simulink model "OFDM_Rx_HW"  (R2020a)
settings: Solver=FixedStepDiscrete  StartTime=0.0  StopTime=inf  RelTol=1e-3
InitFcn:
  | % Set parameters
  | fs = 1e6;
  | 
  | % Load all required variables
  | load('variables/read_addr_data');
  | load('variables/read_addr_cp');
  | load('variables/read_addr_pream');
  | load('variables/read_addr_rx');
  | load('variables/pilot');
  | load('variables/sc_index');
  | load('variables/LTSfreq');
  | load('variables/STSfreq');
  | load('variables/LTSread');
  | load('variables/STSread');
  | 
  | run ./scripts/rfgen;
undefined symbols (not defined in the file or in its folder): LTSfreq, LTSread, pilot, read_addr_cp, read_addr_data, read_addr_pream, read_addr_rx, sc_index, STSfreq, STSread
libraries: hdlsllib x78, simulink x55, xbsIndex_r4 x22, dspmlti4 x19, dspsigops x6, dsphdlmathfun x3, dsphdlxfrm x2, dsphdlsigops x1, lib_rfsignalgenerator x1
(part 1 of 4)
settings Model: SimulationMode=accelerator  Creator=njb13206  LastModifiedBy=david
settings OptimizationCC: BlockReduction=off  ConditionallyExecuteInputs=off  DefaultParameterBehavior=Inlined
settings DebuggingCC: AlgebraicLoopMsg=error  SingleTaskRateTransMsg=error  IntegerOverflowMsg=none  ParameterPrecisionLossMsg=none  IntegerSaturationMsg=none
settings HardwareCC: ProdBitPerPointer=32  ProdBitPerSizeT=32  ProdBitPerPtrDiffT=32  ProdLargestAtomicFloat=None  ProdIntDivRoundTo=Undefined  ProdEndianess=Unspecified  ProdWordSize=32  ProdHWDeviceType=ASIC/FPGA->ASIC/FPGA  TargetBitPerPointer=64  TargetBitPerSizeT=64  TargetBitPerPtrDiffT=64  TargetLongLongMode=on  TargetIntDivRoundTo=Zero  TargetEndianess=LittleEndian  TargetWordSize=64  TargetHWDeviceType=Custom Processor->MATLAB Host Computer  ProdEqTarget=off

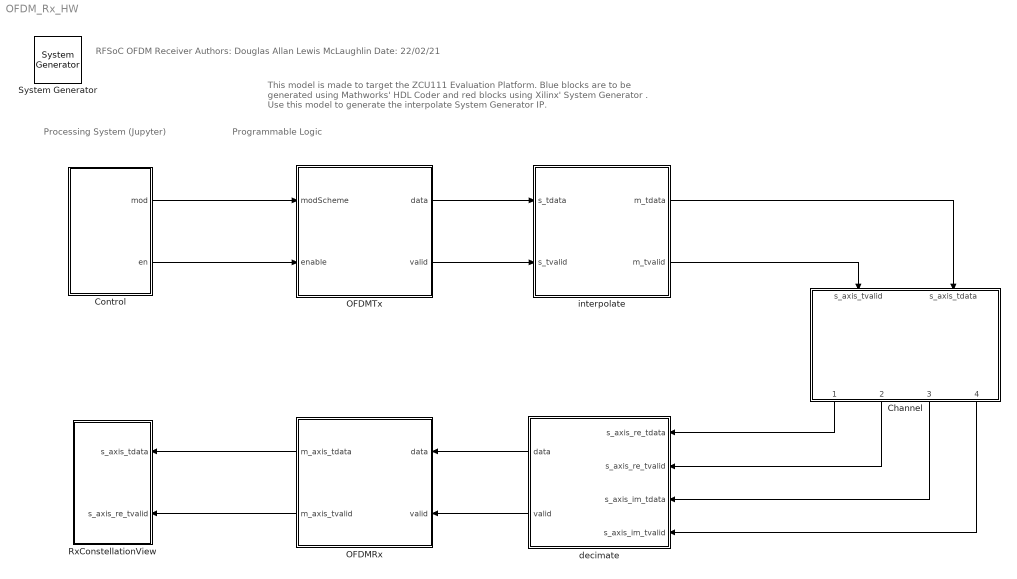
== system OFDM_Rx_HW ==
  note: This model is made to target the ZCU111 Evaluation Platform. Blue blocks are to be generated using Mathworks' HDL Coder and red blocks using Xilinx' System Generator .
      |
      | Use this model to generate the interpolate System Generator IP.
  note: Programmable Logic
  note: Processing System (Jupyter)
  note: RFSoC OFDM Receiver
      | Authors: Douglas Allan
      | Lewis McLaughlin
      | Date: 22/02/21
  " System Generator" : xbsIndex_r4/ System Generator  Tag=genX  xilinxfamily=zynquplusRFSOC  part=xczu28dr  speed=-2-e  package=ffvg1517  synthesis_tool=Vivado  clock_wrapper=Clock Enables  directory=./netlist  proj_type=Vivado  Synth_file=Vivado Synthesis Defaults  Impl_file=Vivado Implementation Defaults  testbench=off  simulink_period=1/256e6  sysclk_period=(1/256e6)*1e9  dcm_input_clock_period=10  incr_netlist=off  trim_vbits=Everywhere in SubSystem  dbl_ovrd=According to Block Masks  core_generation=According to Block Masks  run_coregen=off  deprecated_control=off  eval_field=0  block_type=sysgen
  Channel : Subsystem
  Control : Subsystem  mask{mod_mask=64QAM, en=on}
      mask prompts: mod_mask "Modulation"; en "Enable"
      mask init:
      | % RF Signal Generator
      | if strcmpi(get_param(gcb, 'mod_mask'), 'BPSK')
      |     mod = 0;
      | elseif strcmpi(get_param(gcb, 'mod_mask'), 'QPSK')
      |     mod = 1;
      | elseif strcmpi(get_param(gcb, 'mod_mask'), '8PSK')
      |     mod = 2;
      | elseif strcmpi(get_param(gcb, 'mod_mask'), '16QAM')
      |     mod = 3;
      | elseif strcmpi(get_param(gcb, 'mod_mask'), '32QAM')
      |     mod = 4;
      | elseif strcmpi(get_param(gcb, 'mod_mask'), '64QAM')
      |     mod = 5;
      | elseif strcmpi(get_param(gcb, 'mod_mask'), '128QAM')
      |     mod = 6;
      | elseif strcmpi(get_param(gcb, 'mod_mask'), '256QAM')
      |     mod = 7;
      | elseif strcmpi(get_param(gcb, 'mod_mask'), '512QAM')
      |     mod = 8;
      | elseif strcmpi(get_param(gcb, 'mod_mask'), '1024QAM')
      |     mod = 9;
      | end
      mask TypeOptions mod_mask: BPSK | QPSK | 8PSK | 16QAM | 32QAM | 64QAM | 128QAM | 256QAM | 512QAM | 1024QAM
      mask DialogControl DescGroupVar Prompt: RF Signal Generator
      mask DialogControl DescTextVar Prompt: Exposes parameters the user can control from Jupyter when running on the target.
      mask DialogControl Container3 Prompt: Control
  OFDMRx : Subsystem  TreatAsAtomicUnit=on
  OFDMTx : Subsystem  TreatAsAtomicUnit=on
  RxConstellationView : Subsystem
  decimate : Subsystem
  interpolate : Subsystem
  wires:
  interpolate/1(m_tdata) -> Channel/2(s_axis_tdata)
  OFDMTx/1(data) -> interpolate/1(s_tdata)
  OFDMTx/2(valid) -> interpolate/2(s_tvalid)
  interpolate/2(m_tvalid) -> Channel/1(s_axis_tvalid)
  Channel/4(m_axis_im_tvalid) -> decimate/4(s_axis_im_tvalid)
  OFDMRx/1(m_axis_tdata) -> RxConstellationView/1(s_axis_tdata)
  OFDMRx/2(m_axis_tvalid) -> RxConstellationView/2(s_axis_re_tvalid)
  Channel/1(m00_axis_re_tdata) -> decimate/1(s_axis_re_tdata)
  Channel/2(m_axis_re_tvalid) -> decimate/2(s_axis_re_tvalid)
  Channel/3(m01_axis_im_tdata) -> decimate/3(s_axis_im_tdata)
  decimate/2(valid) -> OFDMRx/2(valid)
  decimate/1(data) -> OFDMRx/1(data)
  Control/1(mod) -> OFDMTx/1(modScheme)
  Control/2(en) -> OFDMTx/2(enable)

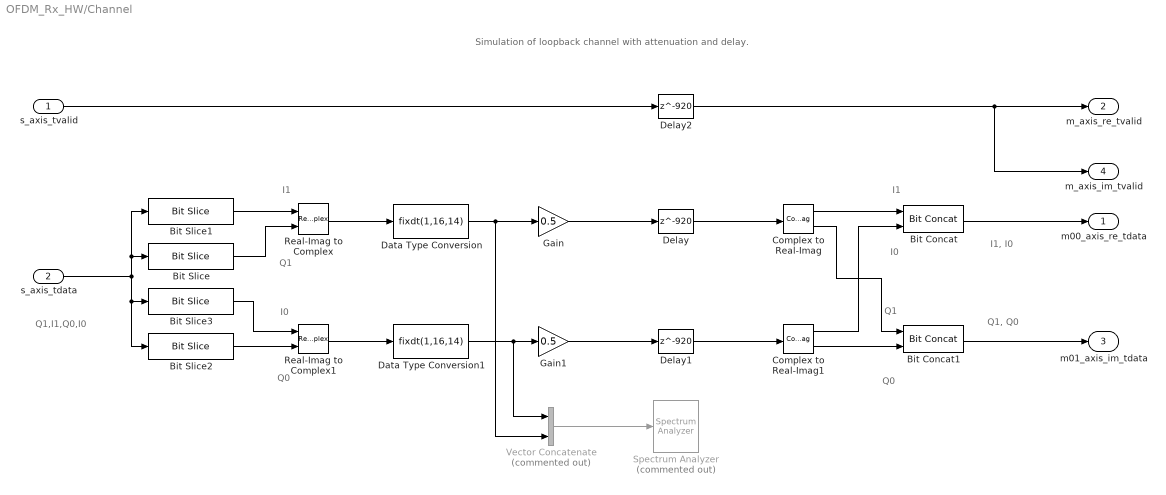
== system OFDM_Rx_HW/Channel ==
  note: Q1, Q0
  note: I1, I0
  note: Q0
  note: I0
  note: Q1
  note: I1
  note: Q1,I1,Q0,I0
  note: Simulation of loopback channel with attenuation and delay.
  note: I1
  note: I0
  note: Q1
  note: Q0
  s_axis_tvalid : Inport
  s_axis_tdata : Inport  Port=2
  Bit Concat : hdlsllib/Logic and Bit Operations/Bit Concat  numInputs=2
  Bit Concat1 : hdlsllib/Logic and Bit Operations/Bit Concat  numInputs=2
  Bit Slice : hdlsllib/Logic and Bit Operations/Bit Slice  lidx=63  ridx=48
      settings: SourceProductBaseCode=SL
  Bit Slice1 : hdlsllib/Logic and Bit Operations/Bit Slice  lidx=47  ridx=32
      settings: SourceProductBaseCode=SL
  Bit Slice2 : hdlsllib/Logic and Bit Operations/Bit Slice  lidx=31  ridx=16
      settings: SourceProductBaseCode=SL
  Bit Slice3 : hdlsllib/Logic and Bit Operations/Bit Slice  lidx=15  ridx=0
      settings: SourceProductBaseCode=SL
  Complex to Real-Imag : ComplexToRealImag
  Complex to Real-Imag1 : ComplexToRealImag
  Data Type Conversion : DataTypeConversion  OutDataTypeStr=fixdt(1,16,14)  ConvertRealWorld=Stored Integer (SI)
  Data Type Conversion1 : DataTypeConversion  OutDataTypeStr=fixdt(1,16,14)  ConvertRealWorld=Stored Integer (SI)
  Delay : Delay  DelayLength=920
  Delay1 : Delay  DelayLength=920
  Delay2 : Delay  DelayLength=920
  Gain : Gain  Gain=0.5  ParamDataTypeStr=double  OutDataTypeStr=fixdt(1,16,14)
  Gain1 : Gain  Gain=0.5  ParamDataTypeStr=double  OutDataTypeStr=fixdt(1,16,14)
  Real-Imag to Complex : RealImagToComplex
  Real-Imag to Complex1 : RealImagToComplex
  Spectrum Analyzer : SpectrumAnalyzer  Commented=on
  Vector Concatenate : Concatenate  Commented=on
  m00_axis_re_tdata : Outport  VectorParamsAs1DForOutWhenUnconnected=off
  m_axis_re_tvalid : Outport  Port=2  VectorParamsAs1DForOutWhenUnconnected=off
  m01_axis_im_tdata : Outport  Port=3  VectorParamsAs1DForOutWhenUnconnected=off
  m_axis_im_tvalid : Outport  Port=4  VectorParamsAs1DForOutWhenUnconnected=off
  wires:
  Gain/1 -> Delay/1
  s_axis_tvalid/1 -> Delay2/1
  Delay/1 -> Complex to Real-Imag/1
  s_axis_tdata/1 -> Bit Slice1/1, Bit Slice/1, Bit Slice2/1, Bit Slice3/1
  Delay1/1 -> Complex to Real-Imag1/1
  Gain1/1 -> Delay1/1
  Bit Concat/1 -> m00_axis_re_tdata/1
  Bit Concat1/1 -> m01_axis_im_tdata/1
  Bit Slice/1 -> Real-Imag to Complex/2
  Bit Slice1/1 -> Real-Imag to Complex/1
  Bit Slice2/1 -> Real-Imag to Complex1/2
  Bit Slice3/1 -> Real-Imag to Complex1/1
  Real-Imag to Complex/1 -> Data Type Conversion/1
  Real-Imag to Complex1/1 -> Data Type Conversion1/1
  Complex to Real-Imag1/1 -> Bit Concat/2
  Complex to Real-Imag/1 -> Bit Concat/1
  Complex to Real-Imag1/2 -> Bit Concat1/2
  Complex to Real-Imag/2 -> Bit Concat1/1
  Data Type Conversion/1 -> Vector Concatenate/2, Gain/1
  Data Type Conversion1/1 -> Vector Concatenate/1, Gain1/1
  Delay2/1 -> m_axis_re_tvalid/1, m_axis_im_tvalid/1
  Vector Concatenate/1 -> Spectrum Analyzer/1

== system OFDM_Rx_HW/Control ==
  Constant2 : Constant  Value=en  OutDataTypeStr=boolean  SampleTime=1/(fs)
  Constant7 : Constant  Value=mod  VectorParams1D=off  OutDataTypeStr=uint32  SampleTime=1/(fs)
  Delay : Delay  DelayLength=randi(10)
  Delay3 : Delay  DelayLength=randi(10)
  mod : Outport  VectorParamsAs1DForOutWhenUnconnected=off
  en : Outport  Port=2  VectorParamsAs1DForOutWhenUnconnected=off
  wires:
  Constant2/1 -> Delay3/1
  Constant7/1 -> Delay/1
  Delay/1 -> mod/1
  Delay3/1 -> en/1

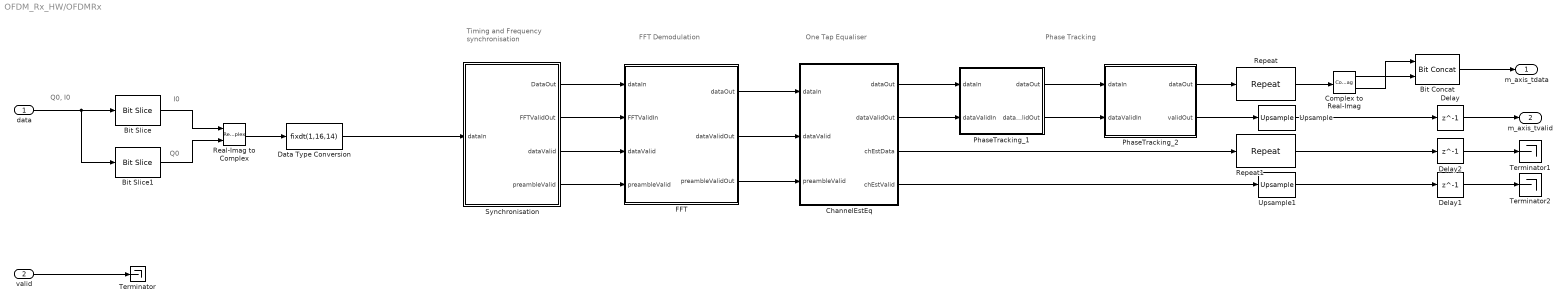
== system OFDM_Rx_HW/OFDMRx ==
  note: Phase Tracking
  note: One Tap Equaliser
  note: FFT Demodulation
  note: Timing and Frequency
      | synchronisation
  note: Q0, I0
  note: I0
  note: Q0
  data : Inport
  valid : Inport  Port=2
  Bit Concat : hdlsllib/Logic and Bit Operations/Bit Concat  numInputs=2
  Bit Slice : hdlsllib/Logic and Bit Operations/Bit Slice  lidx=15  ridx=0
      settings: SourceProductBaseCode=SL
  Bit Slice1 : hdlsllib/Logic and Bit Operations/Bit Slice  lidx=31  ridx=16
      settings: SourceProductBaseCode=SL
  ChannelEstEq : Subsystem
  Complex to Real-Imag : ComplexToRealImag
  Data Type Conversion : DataTypeConversion  OutDataTypeStr=fixdt(1,16,14)  ConvertRealWorld=Stored Integer (SI)
  Delay : Delay  DelayLength=1
  Delay1 : Delay  DelayLength=1
  Delay2 : Delay  DelayLength=1
  FFT : Subsystem
  PhaseTracking_1 : Subsystem
  PhaseTracking_2 : Subsystem
  Real-Imag to Complex : RealImagToComplex
  Repeat : dspsigops/Repeat  N=256  InputProcessing=Columns as channels (frame based)  RateOptions=Allow multirate processing  ic=0  mode=Unused parameter value
  Repeat1 : dspsigops/Repeat  N=256  InputProcessing=Columns as channels (frame based)  RateOptions=Allow multirate processing  ic=0  mode=Unused parameter value
  Synchronisation : Subsystem
  Terminator : Terminator
  Terminator1 : Terminator
  Terminator2 : Terminator
  Upsample : dspsigops/Upsample  N=256  phase=5  RateOptions=Allow multirate processing  ic=0  mode=Unused parameter value
  Upsample1 : dspsigops/Upsample  N=256  phase=5  RateOptions=Allow multirate processing  ic=0  mode=Unused parameter value
  m_axis_tdata : Outport  VectorParamsAs1DForOutWhenUnconnected=off
  m_axis_tvalid : Outport  Port=2  VectorParamsAs1DForOutWhenUnconnected=off
  wires:
  Delay/1 -> m_axis_tvalid/1
  Upsample/1 -> Delay/1
  valid/1 -> Terminator/1
  data/1 -> Bit Slice/1, Bit Slice1/1
  Bit Slice1/1 -> Real-Imag to Complex/2
  Bit Slice/1 -> Real-Imag to Complex/1
  Bit Concat/1 -> m_axis_tdata/1
  Complex to Real-Imag/1 -> Bit Concat/2
  Complex to Real-Imag/2 -> Bit Concat/1
  Repeat/1 -> Complex to Real-Imag/1
  PhaseTracking_2/2(validOut) -> Upsample/1
  PhaseTracking_2/1(dataOut) -> Repeat/1
  Data Type Conversion/1 -> Synchronisation/1(dataIn)
  Real-Imag to Complex/1 -> Data Type Conversion/1
  FFT/1(dataOut) -> ChannelEstEq/1(dataIn)
  FFT/3(preambleValidOut) -> ChannelEstEq/3(preambleValid)
  FFT/2(dataValidOut) -> ChannelEstEq/2(dataValid)
  Synchronisation/1(DataOut) -> FFT/1(dataIn)
  Synchronisation/2(FFTValidOut) -> FFT/2(FFTValidIn)
  Synchronisation/3(dataValid) -> FFT/3(dataValid)
  Synchronisation/4(preambleValid) -> FFT/4(preambleValid)
  ChannelEstEq/1(dataOut) -> PhaseTracking_1/1(dataIn)
  ChannelEstEq/2(dataValidOut) -> PhaseTracking_1/2(dataValidIn)
  PhaseTracking_1/1(dataOut) -> PhaseTracking_2/1(dataIn)
  PhaseTracking_1/2(dataValidOut) -> PhaseTracking_2/2(dataValidIn)
  Upsample1/1 -> Delay1/1
  ChannelEstEq/4(chEstValid) -> Upsample1/1
  ChannelEstEq/3(chEstData) -> Repeat1/1
  Repeat1/1 -> Delay2/1
  Delay2/1 -> Terminator1/1
  Delay1/1 -> Terminator2/1

== system OFDM_Rx_HW/OFDMTx ==
  note: Generate random integers, M-QAM symbol mapping and sub-carrier
      | mapping.
  note: Add Cyclic Prefix
  note: Create OFDM symbols using
      | IFFT
  modScheme : Inport
  enable : Inport  Port=2
  Bit Concat : hdlsllib/Logic and Bit Operations/Bit Concat  numInputs=2
  Bit Slice : hdlsllib/Logic and Bit Operations/Bit Slice  lidx=0  ridx=0
      settings: SourceProductBaseCode=SL
  CPAdd : Subsystem
  Complex to Real-Imag : ComplexToRealImag
  Constant : Constant  OutDataTypeStr=boolean  SampleTime=1/fs
  ControlSignalGenerator : Subsystem
  Data Type Conversion : DataTypeConversion  OutDataTypeStr=uint16  ConvertRealWorld=Stored Integer (SI)
  Data Type Conversion1 : DataTypeConversion  OutDataTypeStr=uint16  ConvertRealWorld=Stored Integer (SI)
  Data Type Conversion2 : DataTypeConversion  OutDataTypeStr=boolean  ConvertRealWorld=Stored Integer (SI)
  DataGenerator : Subsystem
  IFFT : Subsystem
  SCMapper : Subsystem
  Terminator : Terminator
  data : Outport  VectorParamsAs1DForOutWhenUnconnected=off
  valid : Outport  Port=2  VectorParamsAs1DForOutWhenUnconnected=off
  wires:
  Bit Slice/1 -> Data Type Conversion2/1
  enable/1 -> Bit Slice/1
  Data Type Conversion/1 -> Bit Concat/2
  Data Type Conversion1/1 -> Bit Concat/1
  Complex to Real-Imag/2 -> Data Type Conversion1/1
  Complex to Real-Imag/1 -> Data Type Conversion/1
  Bit Concat/1 -> data/1
  modScheme/1 -> DataGenerator/1(modScheme)
  DataGenerator/1(dataOut) -> SCMapper/1(dataIn)
  DataGenerator/2(preambValOut) -> SCMapper/2(preambValid)
  DataGenerator/3(dataValidOut) -> SCMapper/3(dataValid)
  SCMapper/1(dataOut) -> IFFT/1(dataIn)
  SCMapper/2(preambValidOut) -> IFFT/2(preambleValidIn)
  SCMapper/3(dataValidOut) -> IFFT/3("dataValidIn ")
  IFFT/1(dataOut) -> CPAdd/1(dataIn)
  IFFT/2(preambValidOut) -> CPAdd/2(preambValid)
  IFFT/3(dataValidOut) -> CPAdd/3(dataValid)
  CPAdd/1(dataOut) -> Complex to Real-Imag/1
  ControlSignalGenerator/1(dataValid) -> DataGenerator/2(dataValid)
  ControlSignalGenerator/2(preambleValid) -> DataGenerator/3(preambleValid)
  ControlSignalGenerator/3(dataReady) -> DataGenerator/4(dataReady)
  ControlSignalGenerator/4(PilotValid) -> DataGenerator/5(pilotValid)
  Data Type Conversion2/1 -> ControlSignalGenerator/1(enable)
  Constant/1 -> valid/1
  DataGenerator/4(symValidOut) -> Terminator/1

== system OFDM_Rx_HW/RxConstellationView ==
  s_axis_tdata : Inport
  s_axis_re_tvalid : Inport  Port=2
  Bit Slice : hdlsllib/Logic and Bit Operations/Bit Slice  lidx=15  ridx=0
      settings: SourceProductBaseCode=SL
  Bit Slice1 : hdlsllib/Logic and Bit Operations/Bit Slice  lidx=31  ridx=16
      settings: SourceProductBaseCode=SL
  Constant : Constant  Value=NaN + 1i*NaN  OutDataTypeStr=double  SampleTime=-1
  Constellation Diagram : ConstellationDiagram
  Data Type Conversion : DataTypeConversion  OutDataTypeStr=fixdt(1,16,14)  ConvertRealWorld=Stored Integer (SI)
  Real-Imag to Complex : RealImagToComplex
  Switch : Switch  Criteria=u2 ~= 0
  wires:
  Switch/1 -> Constellation Diagram/1
  Constant/1 -> Switch/3
  s_axis_re_tvalid/1 -> Switch/2
  Real-Imag to Complex/1 -> Data Type Conversion/1
  Bit Slice/1 -> Real-Imag to Complex/1
  s_axis_tdata/1 -> Bit Slice1/1, Bit Slice/1
  Bit Slice1/1 -> Real-Imag to Complex/2
  Data Type Conversion/1 -> Switch/1

== system OFDM_Rx_HW/decimate ==
  s_axis_re_tdata : Inport
  s_axis_re_tvalid : Inport  Port=2
  s_axis_im_tdata : Inport  Port=3
  s_axis_im_tvalid : Inport  Port=4
  Decimator : Subsystem
  Terminator : Terminator
  Terminator1 : Terminator
  Unique Decimation : Subsystem  Variant=on  VariantControlMode=Label  VariantControl=Choice  LabelModeActiveChoice=SystemGenerator
  data : Outport
  valid : Outport  Port=2
  wires:
  s_axis_im_tvalid/1 -> Terminator/1
  s_axis_re_tvalid/1 -> Terminator1/1
  s_axis_re_tdata/1 -> Decimator/1(Real In)
  s_axis_im_tdata/1 -> Decimator/2(Imag In)
  Decimator/1(Real Out) -> Unique Decimation/1(Real In)
  Decimator/2(Imag Out) -> Unique Decimation/2(Imag In)
  Decimator/3(Valid Real Out) -> Unique Decimation/3(Valid Real In)
  Decimator/4(Valid Imag Out) -> Unique Decimation/4(Valid Imag In)
  Unique Decimation/1(Data) -> data/1
  Unique Decimation/2(Valid) -> valid/1

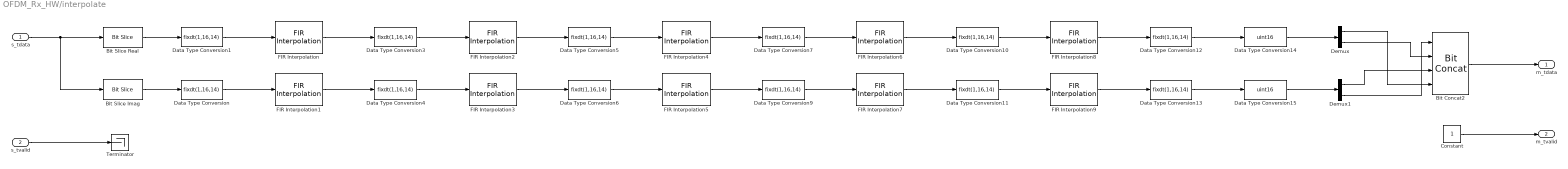
== system OFDM_Rx_HW/interpolate ==
  s_tdata : Inport
  s_tvalid : Inport  Port=2
  Bit Concat2 : hdlsllib/Logic and Bit Operations/Bit Concat  numInputs=4
  Bit Slice Imag : hdlsllib/Logic and Bit Operations/Bit Slice  lidx=31  ridx=16
      settings: SourceProductBaseCode=SL
  Bit Slice Real : hdlsllib/Logic and Bit Operations/Bit Slice  lidx=15  ridx=0
      settings: SourceProductBaseCode=SL
  Constant : Constant  OutDataTypeStr=boolean  SampleTime=1/256e6
  Data Type Conversion : DataTypeConversion  OutDataTypeStr=fixdt(1,16,14)  ConvertRealWorld=Stored Integer (SI)
  Data Type Conversion1 : DataTypeConversion  OutDataTypeStr=fixdt(1,16,14)  ConvertRealWorld=Stored Integer (SI)
  Data Type Conversion{3..7,9..13} (10 alike) : DataTypeConversion  OutDataTypeStr=fixdt(1,16,14)  RndMeth=Round  SaturateOnIntegerOverflow=on
  Data Type Conversion14 : DataTypeConversion  OutDataTypeStr=uint16  ConvertRealWorld=Stored Integer (SI)
  Data Type Conversion15 : DataTypeConversion  OutDataTypeStr=uint16  ConvertRealWorld=Stored Integer (SI)
  Demux : Demux  Outputs=2
  Demux1 : Demux  Outputs=2
  FIR Interpolation : dspmlti4/FIR Interpolation  FilterSource=Dialog parameters  PrivateCoeffs=0  h=interpolation_single.getFilters.Stage1.Numerator  L=2  FilterObject=FINTERP  framing=Allow multirate processing  outputBufInitCond=0  roundingMode=Floor  overflowMode=off  firstCoeffDataTypeStr=Inherit: Same word length as input  firstCoeffMin=[]  firstCoeffMax=[]  firstCoeffLastDataTypeStr=Inherit: Same word length as input  outputDataTypeStr=Inherit: Same as product output  outputMin=[]  outputMax=[]  outputLastDataTypeStr=Inherit: Same as product output
  FIR Interpolation1 : dspmlti4/FIR Interpolation  FilterSource=Dialog parameters  PrivateCoeffs=0  h=interpolation_single.getFilters.Stage1.Numerator  L=2  FilterObject=FINTERP  framing=Allow multirate processing  outputBufInitCond=0  roundingMode=Floor  overflowMode=off  firstCoeffDataTypeStr=Inherit: Same word length as input  firstCoeffMin=[]  firstCoeffMax=[]  firstCoeffLastDataTypeStr=Inherit: Same word length as input  outputDataTypeStr=Inherit: Same as product output  outputMin=[]  outputMax=[]  outputLastDataTypeStr=Inherit: Same as product output
  FIR Interpolation2 : dspmlti4/FIR Interpolation  FilterSource=Dialog parameters  PrivateCoeffs=0  h=interpolation_single.getFilters.Stage2.Numerator  L=2  FilterObject=FINTERP  framing=Allow multirate processing  outputBufInitCond=0  roundingMode=Floor  overflowMode=off  firstCoeffDataTypeStr=Inherit: Same word length as input  firstCoeffMin=[]  firstCoeffMax=[]  firstCoeffLastDataTypeStr=Inherit: Same word length as input  outputDataTypeStr=Inherit: Same as product output  outputMin=[]  outputMax=[]  outputLastDataTypeStr=Inherit: Same as product output
  FIR Interpolation3 : dspmlti4/FIR Interpolation  FilterSource=Dialog parameters  PrivateCoeffs=0  h=interpolation_single.getFilters.Stage2.Numerator  L=2  FilterObject=FINTERP  framing=Allow multirate processing  outputBufInitCond=0  roundingMode=Floor  overflowMode=off  firstCoeffDataTypeStr=Inherit: Same word length as input  firstCoeffMin=[]  firstCoeffMax=[]  firstCoeffLastDataTypeStr=Inherit: Same word length as input  outputDataTypeStr=Inherit: Same as product output  outputMin=[]  outputMax=[]  outputLastDataTypeStr=Inherit: Same as product output
  FIR Interpolation4 : dspmlti4/FIR Interpolation  FilterSource=Dialog parameters  PrivateCoeffs=0  h=interpolation_single.getFilters.Stage3.Numerator  L=4  FilterObject=FINTERP  framing=Allow multirate processing  outputBufInitCond=0  roundingMode=Floor  overflowMode=off  firstCoeffDataTypeStr=Inherit: Same word length as input  firstCoeffMin=[]  firstCoeffMax=[]  firstCoeffLastDataTypeStr=Inherit: Same word length as input  outputDataTypeStr=Inherit: Same as product output  outputMin=[]  outputMax=[]  outputLastDataTypeStr=Inherit: Same as product output
  FIR Interpolation5 : dspmlti4/FIR Interpolation  FilterSource=Dialog parameters  PrivateCoeffs=0  h=interpolation_single.getFilters.Stage3.Numerator  L=4  FilterObject=FINTERP  framing=Allow multirate processing  outputBufInitCond=0  roundingMode=Floor  overflowMode=off  firstCoeffDataTypeStr=Inherit: Same word length as input  firstCoeffMin=[]  firstCoeffMax=[]  firstCoeffLastDataTypeStr=Inherit: Same word length as input  outputDataTypeStr=Inherit: Same as product output  outputMin=[]  outputMax=[]  outputLastDataTypeStr=Inherit: Same as product output
  FIR Interpolation6 : dspmlti4/FIR Interpolation  FilterSource=Dialog parameters  PrivateCoeffs=0  h=interpolation_single.getFilters.Stage4.Numerator  L=16  FilterObject=FINTERP  framing=Allow multirate processing  outputBufInitCond=0  roundingMode=Floor  overflowMode=off  firstCoeffDataTypeStr=Inherit: Same word length as input  firstCoeffMin=[]  firstCoeffMax=[]  firstCoeffLastDataTypeStr=Inherit: Same word length as input  outputDataTypeStr=Inherit: Same as product output  outputMin=[]  outputMax=[]  outputLastDataTypeStr=Inherit: Same as product output
  FIR Interpolation7 : dspmlti4/FIR Interpolation  FilterSource=Dialog parameters  PrivateCoeffs=0  h=interpolation_single.getFilters.Stage4.Numerator  L=16  FilterObject=FINTERP  framing=Allow multirate processing  outputBufInitCond=0  roundingMode=Floor  overflowMode=off  firstCoeffDataTypeStr=Inherit: Same word length as input  firstCoeffMin=[]  firstCoeffMax=[]  firstCoeffLastDataTypeStr=Inherit: Same word length as input  outputDataTypeStr=Inherit: Same as product output  outputMin=[]  outputMax=[]  outputLastDataTypeStr=Inherit: Same as product output
  FIR Interpolation8 : dspmlti4/FIR Interpolation  FilterSource=Dialog parameters  PrivateCoeffs=0  h=interpolation_ssr.Numerator  L=2  FilterObject=FINTERP  InputProcessing=Columns as channels (frame based)  framing=Enforce single-rate processing  outputBufInitCond=0  roundingMode=Floor  overflowMode=off  firstCoeffDataTypeStr=Inherit: Same word length as input  firstCoeffMin=[]  firstCoeffMax=[]  firstCoeffLastDataTypeStr=Inherit: Same word length as input  outputDataTypeStr=Inherit: Same as product output  outputMin=[]  outputMax=[]  outputLastDataTypeStr=Inherit: Same as product output
  FIR Interpolation9 : dspmlti4/FIR Interpolation  FilterSource=Dialog parameters  PrivateCoeffs=0  h=interpolation_ssr.Numerator  L=2  FilterObject=FINTERP  InputProcessing=Columns as channels (frame based)  framing=Enforce single-rate processing  outputBufInitCond=0  roundingMode=Floor  overflowMode=off  firstCoeffDataTypeStr=Inherit: Same word length as input  firstCoeffMin=[]  firstCoeffMax=[]  firstCoeffLastDataTypeStr=Inherit: Same word length as input  outputDataTypeStr=Inherit: Same as product output  outputMin=[]  outputMax=[]  outputLastDataTypeStr=Inherit: Same as product output
  Terminator : Terminator
  m_tdata : Outport
  m_tvalid : Outport  Port=2
  wires:
  Constant/1 -> m_tvalid/1
  Bit Concat2/1 -> m_tdata/1
  s_tdata/1 -> Bit Slice Imag/1, Bit Slice Real/1
  s_tvalid/1 -> Terminator/1
  Bit Slice Real/1 -> Data Type Conversion1/1
  Bit Slice Imag/1 -> Data Type Conversion/1
  Data Type Conversion/1 -> FIR Interpolation1/1
  Data Type Conversion1/1 -> FIR Interpolation/1
  FIR Interpolation/1 -> Data Type Conversion3/1
  FIR Interpolation1/1 -> Data Type Conversion4/1
  Data Type Conversion3/1 -> FIR Interpolation2/1
  Data Type Conversion4/1 -> FIR Interpolation3/1
  FIR Interpolation2/1 -> Data Type Conversion5/1
  FIR Interpolation3/1 -> Data Type Conversion6/1
  Data Type Conversion5/1 -> FIR Interpolation4/1
  Data Type Conversion6/1 -> FIR Interpolation5/1
  FIR Interpolation5/1 -> Data Type Conversion9/1
  FIR Interpolation4/1 -> Data Type Conversion7/1
  FIR Interpolation7/1 -> Data Type Conversion11/1
  Data Type Conversion7/1 -> FIR Interpolation6/1
  Data Type Conversion9/1 -> FIR Interpolation7/1
  FIR Interpolation6/1 -> Data Type Conversion10/1
  Data Type Conversion10/1 -> FIR Interpolation8/1
  Data Type Conversion11/1 -> FIR Interpolation9/1
  FIR Interpolation9/1 -> Data Type Conversion13/1
  FIR Interpolation8/1 -> Data Type Conversion12/1
  Data Type Conversion12/1 -> Data Type Conversion14/1
  Data Type Conversion13/1 -> Data Type Conversion15/1
  Data Type Conversion14/1 -> Demux/1
  Data Type Conversion15/1 -> Demux1/1
  Demux/1 -> Bit Concat2/4
  Demux1/1 -> Bit Concat2/3
  Demux/2 -> Bit Concat2/2
  Demux1/2 -> Bit Concat2/1

== system OFDM_Rx_HW/OFDMRx/ChannelEstEq ==
  dataIn : Inport
  dataValid : Inport  Port=2
  preambleValid : Inport  Port=3
  Bit Concat1 : hdlsllib/Logic and Bit Operations/Bit Concat  numInputs=2
  ChannelEstimate : Subsystem
  Complex to Real-Imag1 : ComplexToRealImag
  Data Type Conversion1 : DataTypeConversion  OutDataTypeStr=fixdt(1,16,14)
  Data Type Conversion3 : DataTypeConversion  OutDataTypeStr=uint16  ConvertRealWorld=Stored Integer (SI)
  Data Type Conversion4 : DataTypeConversion  OutDataTypeStr=uint16  ConvertRealWorld=Stored Integer (SI)
  Delay : Delay  DelayLength=6
  Equalise : Subsystem
  dataOut : Outport  VectorParamsAs1DForOutWhenUnconnected=off
  dataValidOut : Outport  Port=2  VectorParamsAs1DForOutWhenUnconnected=off
  chEstData : Outport  Port=3  VectorParamsAs1DForOutWhenUnconnected=off
  chEstValid : Outport  Port=4  VectorParamsAs1DForOutWhenUnconnected=off
  wires:
  ChannelEstimate/1(chEstOut) -> Equalise/2(chEstIn), Data Type Conversion1/1
  Delay/1 -> Equalise/1(dataInEq)
  dataIn/1 -> ChannelEstimate/1(dataIn), Delay/1
  preambleValid/1 -> ChannelEstimate/2(preambleValid)
  dataValid/1 -> ChannelEstimate/3(dataValidIn)
  Equalise/1(dataOutEq) -> dataOut/1
  Equalise/2(dataValidOut) -> dataValidOut/1
  ChannelEstimate/2(dataValidOut) -> chEstValid/1, Equalise/3(dataValidIn)
  Data Type Conversion4/1 -> Bit Concat1/1
  Bit Concat1/1 -> chEstData/1
  Data Type Conversion3/1 -> Bit Concat1/2
  Complex to Real-Imag1/2 -> Data Type Conversion4/1
  Complex to Real-Imag1/1 -> Data Type Conversion3/1
  Data Type Conversion1/1 -> Complex to Real-Imag1/1

== system OFDM_Rx_HW/OFDMRx/FFT ==
  dataIn : Inport
  FFTValidIn : Inport  Port=2
  dataValid : Inport  Port=3
  preambleValid : Inport  Port=4
  Delay1 : Delay  DelayLength=173
  Delay2 : Delay  DelayLength=173
  FFT HDL Optimized : dsphdlxfrm/FFT HDL Optimized  FFTLength=64  Architecture=Streaming Radix 2^2  ComplexMultiplication=Use 4 multipliers and 2 adders  BitReversedOutput=off  BitReversedInput=off  Normalize=off  SimulateUsing=Code generation  RoundingMethod=Floor  ResetInputPort=off  StartOutputPort=off  EndOutputPort=off
      settings: SourceProductBaseCode=DS
  Terminator : Terminator
  dataOut : Outport  VectorParamsAs1DForOutWhenUnconnected=off
  dataValidOut : Outport  Port=2  VectorParamsAs1DForOutWhenUnconnected=off
  preambleValidOut : Outport  Port=3  VectorParamsAs1DForOutWhenUnconnected=off
  wires:
  FFTValidIn/1 -> FFT HDL Optimized/2
  dataIn/1 -> FFT HDL Optimized/1
  Delay2/1 -> dataValidOut/1
  Delay1/1 -> preambleValidOut/1
  FFT HDL Optimized/1 -> dataOut/1
  FFT HDL Optimized/2 -> Terminator/1
  dataValid/1 -> Delay2/1
  preambleValid/1 -> Delay1/1

== system OFDM_Rx_HW/OFDMRx/PhaseTracking_1 ==
  note: Phase Tracking Stage 1: Track linear phase error which occurs due to sampling phase/frequency offsets. The implemented algorithm
      | estimates the gradient of the linear phase error using pilot sub-carriers.
  dataIn : Inport
  dataValidIn : Inport  Port=2
  CordicRotate : Subsystem
  DataArrange : Subsystem
  "GradientEstimate " : Subsystem
  PhaseErrorEst : Subsystem
  PilotCtrlGen : Subsystem
  dataOut : Outport
  dataValidOut : Outport  Port=2
  wires:
  CordicRotate/2(dataValidOut) -> dataValidOut/1
  PhaseErrorEst/3(dataValidOut) -> CordicRotate/3(dataValidIn)
  PhaseErrorEst/2(PhaseOut) -> CordicRotate/2(PhaseInRotate)
  PhaseErrorEst/1(dataOut) -> CordicRotate/1(DataInRotate)
  "GradientEstimate "/1(dataOut) -> PhaseErrorEst/1(dataIn)
  "GradientEstimate "/2(gradientOut) -> PhaseErrorEst/2(gradientIn)
  "GradientEstimate "/3(dataValidOut) -> PhaseErrorEst/3(dataValidIn)
  CordicRotate/1("DataOutRotate  ") -> dataOut/1
  dataIn/1 -> DataArrange/1(dataIn)
  dataValidIn/1 -> DataArrange/2(dataValidIn)
  DataArrange/1(dataOut) -> PilotCtrlGen/1(dataIn)
  DataArrange/2(dataValidOut) -> PilotCtrlGen/2(validIn)
  PilotCtrlGen/1(dataOut) -> "GradientEstimate "/1(dataIn)
  PilotCtrlGen/2(pilotOut) -> "GradientEstimate "/2(pilotIn)
  PilotCtrlGen/3(pilotEnd) -> "GradientEstimate "/3(PilotEnd)
  PilotCtrlGen/4(dataValid) -> "GradientEstimate "/4(dataValid)

== system OFDM_Rx_HW/OFDMRx/PhaseTracking_2 ==
  note: Phase Tracking Stage 2:  Track Common Phase Error (CPE) from symbol to symbol.
      | CPE is caused by residual frequency offset and phase noise effects.
  dataIn : Inport
  dataValidIn : Inport  Port=2
  CordicRotate : Subsystem
  PhaseEst : Subsystem
  PilotCtrlGen : Subsystem
  dataOut : Outport  VectorParamsAs1DForOutWhenUnconnected=off
  validOut : Outport  Port=2  VectorParamsAs1DForOutWhenUnconnected=off
  wires:
  PilotCtrlGen/1(dataOut) -> PhaseEst/1(dataIn)
  PilotCtrlGen/2(pilotOut) -> PhaseEst/2(PilotIn)
  PilotCtrlGen/3(PilotEnd) -> PhaseEst/3(pilotEnd)
  PilotCtrlGen/4(dataValid) -> PhaseEst/4(dataValid)
  PhaseEst/1(dataOut) -> CordicRotate/1(DataIn)
  PhaseEst/2(phaseOut) -> CordicRotate/2(PhaseIn)
  PhaseEst/3(validOut) -> CordicRotate/3(validIn)
  CordicRotate/1("DataOut  ") -> dataOut/1
  CordicRotate/2(validOut) -> validOut/1
  dataIn/1 -> PilotCtrlGen/1(dataIn)
  dataValidIn/1 -> PilotCtrlGen/2(ValidIn)

== system OFDM_Rx_HW/OFDMRx/Synchronisation ==
  dataIn : Inport
  CoarseFreqCorr : Subsystem
  ControlSigGen : Subsystem
  Delay : Subsystem
  Delay1 : Delay  DelayLength=22  InputProcessing=Columns as channels (frame based)
  Delay2 : Delay  InputProcessing=Columns as channels (frame based)
  Delay4 : Delay  DelayLength=1  InputProcessing=Columns as channels (frame based)
  FrameDetect : Subsystem
  "SchmidlCoxMetric " : Subsystem
  DataOut : Outport  VectorParamsAs1DForOutWhenUnconnected=off
  FFTValidOut : Outport  Port=2  VectorParamsAs1DForOutWhenUnconnected=off
  dataValid : Outport  Port=3  VectorParamsAs1DForOutWhenUnconnected=off
  preambleValid : Outport  Port=4  VectorParamsAs1DForOutWhenUnconnected=off
  wires:
  dataIn/1 -> "SchmidlCoxMetric "/1(dataIn), Delay1/1
  ControlSigGen/1(FFTValid) -> FFTValidOut/1
  ControlSigGen/2(dataValid) -> dataValid/1
  ControlSigGen/3(preambleValid) -> preambleValid/1
  Delay1/1 -> Delay2/1
  "SchmidlCoxMetric "/1(left) -> FrameDetect/1(leftIn)
  "SchmidlCoxMetric "/2(right) -> FrameDetect/2(rightIn)
  "SchmidlCoxMetric "/3(phase) -> FrameDetect/3(phaseIn)
  FrameDetect/2(phaseOut) -> CoarseFreqCorr/3(phaseIn)
  Delay2/1 -> CoarseFreqCorr/1(dataIn)
  FrameDetect/1(frameDet) -> CoarseFreqCorr/2(frameDet)
  Delay4/1 -> DataOut/1
  CoarseFreqCorr/2(frameDetOut) -> Delay/2(strobe)
  CoarseFreqCorr/1(dataOut) -> Delay/1(data)
  Delay/2(strobeOut) -> ControlSigGen/1(validIn)
  Delay/1(dataOut) -> Delay4/1

== system OFDM_Rx_HW/OFDMTx/CPAdd ==
  dataIn : Inport
  preambValid : Inport  Port=2
  dataValid : Inport  Port=3
  DataExtend : Subsystem
  LTFExtend : Subsystem
  Mux2 : MATLAB Function  TreatAsAtomicUnit=on
  STFExtend : Subsystem
  dataOut : Outport  VectorParamsAs1DForOutWhenUnconnected=off
  wires:
  preambValid/1 -> LTFExtend/2(preambVal), STFExtend/2(preambVal)
  dataIn/1 -> DataExtend/1(dataIn), LTFExtend/1(data), STFExtend/1(data)
  STFExtend/1(STFExtendOut) -> Mux2/1(sts)
  STFExtend/2(STFValidOut) -> Mux2/2(stsval)
  LTFExtend/1(LTFExtendOut) -> Mux2/3(lts)
  LTFExtend/2(LTFValidOut) -> Mux2/4(ltsval)
  DataExtend/1(dataOut) -> Mux2/5(data)
  DataExtend/2(dataValidOut) -> Mux2/6(dataval)
  Mux2/1(dataOut) -> dataOut/1
  dataValid/1 -> DataExtend/2(dataValid)

== system OFDM_Rx_HW/OFDMTx/ControlSignalGenerator ==
  enable : Inport
  PreamValidGen : Subsystem
  dataReadyGen : Subsystem
  dataValidGen : Subsystem
  pilotValidGen : Subsystem
  dataValid : Outport
  preambleValid : Outport  Port=2
  dataReady : Outport  Port=3
  PilotValid : Outport  Port=4
  wires:
  enable/1 -> dataValidGen/2(enable), PreamValidGen/1(enable)
  dataReadyGen/1(y) -> dataReady/1
  pilotValidGen/1(y) -> PilotValid/1
  PreamValidGen/1(y) -> preambleValid/1, dataValidGen/1(y)
  dataValidGen/1(valOut) -> pilotValidGen/1(enb), dataReadyGen/1(enb), dataValid/1

== system OFDM_Rx_HW/OFDMTx/DataGenerator ==
  modScheme : Inport
  dataValid : Inport  Port=2
  preambleValid : Inport  Port=3
  dataReady : Inport  Port=4
  pilotValid : Inport  Port=5
  Constant : Constant  Value=0  OutDataTypeStr=boolean  SampleTime=1/fs
  Data Multiplexer : MATLAB Function  TreatAsAtomicUnit=on
  LTSfreq : Subsystem
  PilotGen : Subsystem
  RF Signal Generator : lib_rfsignalgenerator/RF Signal Generator  SystemSampleTime=-1  Latency=0  AutoFrameSizeCalculation=off
  STSFreq : Subsystem
  dataOut : Outport  VectorParamsAs1DForOutWhenUnconnected=off
  preambValOut : Outport  Port=2  VectorParamsAs1DForOutWhenUnconnected=off
  dataValidOut : Outport  Port=3  VectorParamsAs1DForOutWhenUnconnected=off
  symValidOut : Outport  Port=4  VectorParamsAs1DForOutWhenUnconnected=off
  wires:
  dataValid/1 -> PilotGen/1(dataValidIn), dataValidOut/1
  preambleValid/1 -> STSFreq/1(preamVal), LTSfreq/1(preambVal), preambValOut/1
  LTSfreq/2(ltsVal) -> Data Multiplexer/8(ltsval)
  LTSfreq/1(ltsFreq) -> Data Multiplexer/7(lts)
  STSFreq/2(stsVal) -> Data Multiplexer/6(stsval)
  STSFreq/1(stsFreq) -> Data Multiplexer/5(sts)
  pilotValid/1 -> PilotGen/2(pilotValidIn), Data Multiplexer/4(pval)
  PilotGen/1(pilotOut) -> Data Multiplexer/3(pilots)
  RF Signal Generator/2 -> Data Multiplexer/1(symbols)
  Data Multiplexer/1(data) -> dataOut/1
  modScheme/1 -> RF Signal Generator/1
  RF Signal Generator/1 -> symValidOut/1
  Constant/1 -> RF Signal Generator/2
  dataReady/1 -> RF Signal Generator/3, Data Multiplexer/2(dataready)

== system OFDM_Rx_HW/OFDMTx/IFFT ==
  dataIn : Inport
  preambleValidIn : Inport  Port=2
  "dataValidIn " : Inport  Port=3
  Delay : Delay  DelayLength=173  InitialCondition=0  UseCircularBuffer=on
  Delay1 : Delay  DelayLength=173  InitialCondition=0  UseCircularBuffer=on
  IFFT HDL Optimized : dsphdlxfrm/IFFT HDL Optimized  FFTLength=64  Architecture=Streaming Radix 2^2  ComplexMultiplication=Use 3 multipliers and 5 adders  BitReversedOutput=off  BitReversedInput=off  Normalize=on  SimulateUsing=Code generation  RoundingMethod=Floor  ResetInputPort=off  StartOutputPort=off  EndOutputPort=off
      settings: SourceProductBaseCode=DS
  IFFTValid : Subsystem
  Terminator : Terminator
  dataOut : Outport  VectorParamsAs1DForOutWhenUnconnected=off
  preambValidOut : Outport  Port=2  VectorParamsAs1DForOutWhenUnconnected=off
  dataValidOut : Outport  Port=3  VectorParamsAs1DForOutWhenUnconnected=off
  wires:
  dataIn/1 -> IFFT HDL Optimized/1
  IFFT HDL Optimized/2 -> Terminator/1
  "dataValidIn "/1 -> IFFTValid/2(dataValid), Delay1/1
  IFFTValid/1(ifftValid) -> IFFT HDL Optimized/2
  preambleValidIn/1 -> IFFTValid/1(preambleValid), Delay/1
  Delay/1 -> preambValidOut/1
  Delay1/1 -> dataValidOut/1
  IFFT HDL Optimized/1 -> dataOut/1

== system OFDM_Rx_HW/OFDMTx/SCMapper ==
  dataIn : Inport
  preambValid : Inport  Port=2
  dataValid : Inport  Port=3
  DataMapper : Subsystem
  Mux2 : MATLAB Function  TreatAsAtomicUnit=on
  PremableMapper : Subsystem
  dataOut : Outport  VectorParamsAs1DForOutWhenUnconnected=off
  preambValidOut : Outport  Port=2  VectorParamsAs1DForOutWhenUnconnected=off
  dataValidOut : Outport  Port=3  VectorParamsAs1DForOutWhenUnconnected=off
  wires:
  PremableMapper/1(preambleShiftOut) -> Mux2/1(preamb)
  PremableMapper/2(preambValOut) -> preambValidOut/1, Mux2/2(preambVal)
  DataMapper/1(dataOut) -> Mux2/3(data)
  DataMapper/2(dataValidOut) -> dataValidOut/1, Mux2/4(dataVal)
  dataIn/1 -> DataMapper/1(dataIn), PremableMapper/1(data)
  preambValid/1 -> PremableMapper/2(preambVal)
  dataValid/1 -> DataMapper/2(dataValid)
  Mux2/1(dataOut) -> dataOut/1

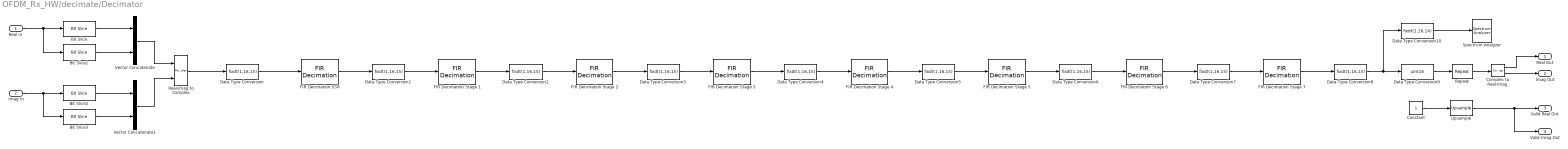
== system OFDM_Rx_HW/decimate/Decimator ==
  Real In : Inport
  Imag In : Inport  Port=2
  Bit Slice : hdlsllib/Logic and Bit Operations/Bit Slice  lidx=15  ridx=0
      settings: SourceProductBaseCode=SL
  Bit Slice1 : hdlsllib/Logic and Bit Operations/Bit Slice  lidx=31  ridx=16
      settings: SourceProductBaseCode=SL
  Bit Slice2 : hdlsllib/Logic and Bit Operations/Bit Slice  lidx=15  ridx=0
      settings: SourceProductBaseCode=SL
  Bit Slice3 : hdlsllib/Logic and Bit Operations/Bit Slice  lidx=31  ridx=16
      settings: SourceProductBaseCode=SL
  Complex to Real-Imag : ComplexToRealImag
  Constant : Constant  OutDataTypeStr=boolean  SampleTime=1/(2e6)
  Data Type Conversion : DataTypeConversion  OutDataTypeStr=fixdt(1,16,15)  ConvertRealWorld=Stored Integer (SI)
  Data Type Conversion{1..8} (8 alike) : DataTypeConversion  OutDataTypeStr=fixdt(1,16,15)  RndMeth=Round  SaturateOnIntegerOverflow=on
  Data Type Conversion10 : DataTypeConversion  OutDataTypeStr=fixdt(1,16,14)  ConvertRealWorld=Stored Integer (SI)
  Data Type Conversion9 : DataTypeConversion  OutDataTypeStr=uint16  ConvertRealWorld=Stored Integer (SI)
  FIR Decimation SSR : dspmlti4/FIR Decimation  FilterSource=Dialog parameters  h=decimation_ssr.Numerator  D=2  filtStruct=Direct form  FilterObject=FDECIM  InputProcessing=Columns as channels (frame based)  framing=Enforce single-rate processing  inputOffset=0  outputBufInitCond=0  roundingMode=Floor  overflowMode=off  firstCoeffDataTypeStr=Inherit: Same word length as input  firstCoeffMin=[]  firstCoeffMax=[]  firstCoeffLastDataTypeStr=Inherit: Same word length as input  outputDataTypeStr=Inherit: Same as product output  outputMin=[]  outputMax=[]  outputLastDataTypeStr=Inherit: Same as product output
  FIR Decimation Stage {1..7} (7 alike) : dspmlti4/FIR Decimation  FilterSource=Dialog parameters  h=decimation_single.Numerator  D=2  filtStruct=Direct form  FilterObject=FDECIM  framing=Enforce single-rate processing  inputOffset=0  outputBufInitCond=0  roundingMode=Floor  overflowMode=off  firstCoeffDataTypeStr=Inherit: Same word length as input  firstCoeffMin=[]  firstCoeffMax=[]  firstCoeffLastDataTypeStr=Inherit: Same word length as input  outputDataTypeStr=Inherit: Same as product output  outputMin=[]  outputMax=[]  outputLastDataTypeStr=Inherit: Same as product output
  Real-Imag to Complex : RealImagToComplex
  Repeat : dspsigops/Repeat  N=128  RateOptions=Allow multirate processing  ic=0  mode=Unused parameter value
  Spectrum Analyzer : SpectrumAnalyzer
  Upsample : dspsigops/Upsample  N=128  phase=0  RateOptions=Allow multirate processing  ic=0  mode=Unused parameter value
  Vector Concatenate : Concatenate
  Vector Concatenate1 : Concatenate
  Real Out : Outport
  Imag Out : Outport  Port=2
  Valid Real Out : Outport  Port=3
  Valid Imag Out : Outport  Port=4
  wires:
  Data Type Conversion4/1 -> FIR Decimation Stage 4/1
  Data Type Conversion5/1 -> FIR Decimation Stage 5/1
  Complex to Real-Imag/1 -> Real Out/1
  FIR Decimation Stage 3/1 -> Data Type Conversion4/1
  Bit Slice3/1 -> Vector Concatenate1/2
  Data Type Conversion/1 -> FIR Decimation SSR/1
  FIR Decimation Stage 4/1 -> Data Type Conversion5/1
  Imag In/1 -> Bit Slice2/1, Bit Slice3/1
  Constant/1 -> Upsample/1
  Bit Slice2/1 -> Vector Concatenate1/1
  Data Type Conversion7/1 -> FIR Decimation Stage 7/1
  FIR Decimation Stage 2/1 -> Data Type Conversion3/1
  Data Type Conversion6/1 -> FIR Decimation Stage 6/1
  Real In/1 -> Bit Slice1/1, Bit Slice/1
  Data Type Conversion8/1 -> Data Type Conversion10/1, Data Type Conversion9/1
  FIR Decimation Stage 7/1 -> Data Type Conversion8/1
  FIR Decimation SSR/1 -> Data Type Conversion1/1
  Bit Slice/1 -> Vector Concatenate/1
  FIR Decimation Stage 5/1 -> Data Type Conversion6/1
  Bit Slice1/1 -> Vector Concatenate/2
  Real-Imag to Complex/1 -> Data Type Conversion/1
  Data Type Conversion3/1 -> FIR Decimation Stage 3/1
  Vector Concatenate/1 -> Real-Imag to Complex/1
  Vector Concatenate1/1 -> Real-Imag to Complex/2
  Complex to Real-Imag/2 -> Imag Out/1
  FIR Decimation Stage 1/1 -> Data Type Conversion2/1
  Data Type Conversion1/1 -> FIR Decimation Stage 1/1
  FIR Decimation Stage 6/1 -> Data Type Conversion7/1
  Data Type Conversion2/1 -> FIR Decimation Stage 2/1
  Repeat/1 -> Complex to Real-Imag/1
  Data Type Conversion9/1 -> Repeat/1
  Upsample/1 -> Valid Imag Out/1, Valid Real Out/1
  Data Type Conversion10/1 -> Spectrum Analyzer/1

== system OFDM_Rx_HW/decimate/Unique Decimation ==
  Real In : Inport
  Imag In : Inport  Port=2
  Valid Real In : Inport  Port=3
  Valid Imag In : Inport  Port=4
  Unique Decimation : Subsystem  VariantControl=SystemGenerator
  Unique Decimation1 : Subsystem  VariantControl=Simulink
  Data : Outport
  Valid : Outport  Port=2

== system OFDM_Rx_HW/OFDMRx/ChannelEstEq/ChannelEstimate ==
  note: Note the preamble symbols do not pass this point.
  note: Write averaged channel estimate to RAM and read out when data is valid
      | for equalisation of successive OFDM symbols.
  note: Get and store the channel estimate using the two
      | repetitions of the L-LTF
  dataIn : Inport
  preambleValid : Inport  Port=2
  dataValidIn : Inport  Port=3
  ChanEst : Subsystem
  Delay : Delay  DelayLength=5
  Delay1 : Delay  DelayLength=5
  Delay2 : Delay  DelayLength=1
  Dual Port RAM1 : hdlsllib/HDL RAMs/Dual Port RAM  ram_size=6
      settings: SourceProductBaseCode=SL
  HDL Counter3 : hdlsllib/Sources/HDL Counter  CountType=Count limited  CountInit=0  CountStep=1  CountMax=63  CountFromType=Initial value  CountFrom=0  CountResetPort=off  CountLoadPort=off  CountEnbPort=on  CountDirPort=off  CountDataType=Unsigned  CountWordLen=6  CountFracLen=0  CountSampTime=1
  Terminator : Terminator
  WriteEnbAddrGen : Subsystem
  chEstOut : Outport  VectorParamsAs1DForOutWhenUnconnected=off
  dataValidOut : Outport  Port=2  VectorParamsAs1DForOutWhenUnconnected=off
  wires:
  HDL Counter3/1 -> Dual Port RAM1/4
  Dual Port RAM1/2 -> chEstOut/1
  Delay2/1 -> dataValidOut/1
  preambleValid/1 -> ChanEst/2(PreambValidIn), Delay/1
  dataIn/1 -> ChanEst/1(ChanEstIn)
  ChanEst/1(ChEstOut) -> Dual Port RAM1/1
  dataValidIn/1 -> Delay1/1
  Delay1/1 -> HDL Counter3/1, Delay2/1
  Delay/1 -> WriteEnbAddrGen/1(In1)
  WriteEnbAddrGen/1(Out1) -> Dual Port RAM1/2
  WriteEnbAddrGen/2(Out2) -> Dual Port RAM1/3
  Dual Port RAM1/1 -> Terminator/1

== system OFDM_Rx_HW/OFDMRx/ChannelEstEq/Equalise ==
  note: Perform a complex division to obtain equalised data symbols.
  dataInEq : Inport
  chEstIn : Inport  Port=2
  dataValidIn : Inport  Port=3
  Abs2 : Subsystem
  Complex Mult : Subsystem
  Delay1 : Delay
  Delay8 : Delay  DelayLength=3
  Divide : Subsystem
  dataOutEq : Outport  VectorParamsAs1DForOutWhenUnconnected=off
  dataValidOut : Outport  Port=2  VectorParamsAs1DForOutWhenUnconnected=off
  wires:
  dataValidIn/1 -> Delay8/1
  chEstIn/1 -> Abs2/1(ChEstIn), Complex Mult/2(In2)
  dataInEq/1 -> Complex Mult/1(In1)
  Complex Mult/1(Out1) -> Divide/1(In1)
  Abs2/1(Out1) -> Divide/2(In2)
  Delay8/1 -> Delay1/1
  Delay1/1 -> dataValidOut/1
  Divide/1(dataOutEq) -> dataOutEq/1

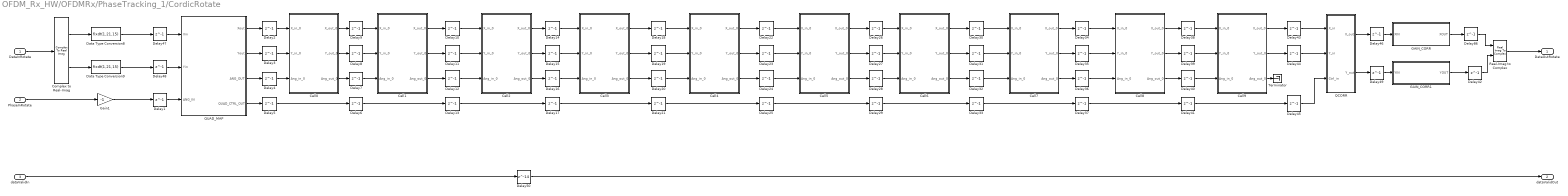
== system OFDM_Rx_HW/OFDMRx/PhaseTracking_1/CordicRotate ==
  DataInRotate : Inport
  PhaseInRotate : Inport  Port=2
  dataValidIn : Inport  Port=3
  Cell0 : Subsystem
  Cell1 : Subsystem
  Cell2 : Subsystem
  Cell3 : Subsystem
  Cell4 : Subsystem
  Cell5 : Subsystem
  Cell6 : Subsystem
  Cell7 : Subsystem
  Cell8 : Subsystem
  Cell9 : Subsystem
  Complex to Real-Imag : ComplexToRealImag
  Data Type Conversion8 : DataTypeConversion  OutDataTypeStr=fixdt(1,21,15)
  Data Type Conversion9 : DataTypeConversion  OutDataTypeStr=fixdt(1,21,15)
  Delay{1..49,86} (50 alike) : Delay  DelayLength=1
  Delay50 : Delay  DelayLength=14
  GAIN_CORR : Subsystem
  GAIN_CORR1 : Subsystem
  Gain1 : Gain  Gain=-1  OutDataTypeStr=fixdt(1,23,20)
  QCORR : Subsystem
  QUAD_MAP : Subsystem
  Real-Imag to Complex : RealImagToComplex
  Terminator : Terminator
  "DataOutRotate  " : Outport  VectorParamsAs1DForOutWhenUnconnected=off
  dataValidOut : Outport  Port=2  VectorParamsAs1DForOutWhenUnconnected=off
  wires:
  Delay50/1 -> dataValidOut/1
  dataValidIn/1 -> Delay50/1
  Gain1/1 -> Delay1/1
  PhaseInRotate/1 -> Gain1/1
  QCORR/1(X_out) -> Delay46/1
  Data Type Conversion9/1 -> Delay48/1
  Data Type Conversion8/1 -> Delay47/1
  Delay45/1 -> QCORR/3(Ctrl_in)
  Delay4/1 -> Cell0/3(Ang_in_0)
  Delay1/1 -> QUAD_MAP/3(ANG_IN)
  QCORR/2(Y_out) -> Delay49/1
  Delay49/1 -> GAIN_CORR1/1(YIN)
  Delay46/1 -> GAIN_CORR/1(XIN)
  Delay44/1 -> QCORR/2(Y_in)
  Delay43/1 -> QCORR/1(X_in)
  Cell9/2(Y_out_0) -> Delay44/1
  Cell9/1(X_out_0) -> Delay43/1
  Delay41/1 -> Delay45/1
  Cell9/3(Ang_out_0) -> Terminator/1
  GAIN_CORR1/1(YOUT) -> Delay42/1
  Cell8/1(X_out_0) -> Delay38/1
  Cell8/2(Y_out_0) -> Delay39/1
  Cell8/3(Ang_out_0) -> Delay40/1
  Delay37/1 -> Delay41/1
  Delay38/1 -> Cell9/1(X_in_0)
  Delay39/1 -> Cell9/2(Y_in_0)
  Delay40/1 -> Cell9/3(Ang_in_0)
  Delay36/1 -> Cell8/3(Ang_in_0)
  Delay35/1 -> Cell8/2(Y_in_0)
  Delay34/1 -> Cell8/1(X_in_0)
  Delay33/1 -> Delay37/1
  Cell7/3(Ang_out_0) -> Delay36/1
  Cell7/2(Y_out_0) -> Delay35/1
  Cell7/1(X_out_0) -> Delay34/1
  Cell6/1(X_out_0) -> Delay30/1
  Cell6/2(Y_out_0) -> Delay31/1
  Cell6/3(Ang_out_0) -> Delay32/1
  Delay29/1 -> Delay33/1
  Delay30/1 -> Cell7/1(X_in_0)
  Delay31/1 -> Cell7/2(Y_in_0)
  Delay32/1 -> Cell7/3(Ang_in_0)
  Delay28/1 -> Cell6/3(Ang_in_0)
  Delay27/1 -> Cell6/2(Y_in_0)
  Delay26/1 -> Cell6/1(X_in_0)
  Delay25/1 -> Delay29/1
  Cell5/3(Ang_out_0) -> Delay28/1
  Cell5/2(Y_out_0) -> Delay27/1
  Cell5/1(X_out_0) -> Delay26/1
  Cell4/1(X_out_0) -> Delay22/1
  Cell4/2(Y_out_0) -> Delay23/1
  Cell4/3(Ang_out_0) -> Delay24/1
  Delay21/1 -> Delay25/1
  Delay22/1 -> Cell5/1(X_in_0)
  Delay23/1 -> Cell5/2(Y_in_0)
  Delay24/1 -> Cell5/3(Ang_in_0)
  Delay20/1 -> Cell4/3(Ang_in_0)
  Delay19/1 -> Cell4/2(Y_in_0)
  Delay18/1 -> Cell4/1(X_in_0)
  Delay17/1 -> Delay21/1
  Cell3/3(Ang_out_0) -> Delay20/1
  Cell3/2(Y_out_0) -> Delay19/1
  Cell3/1(X_out_0) -> Delay18/1
  Cell2/1(X_out_0) -> Delay14/1
  Cell2/2(Y_out_0) -> Delay15/1
  Cell2/3(Ang_out_0) -> Delay16/1
  Delay13/1 -> Delay17/1
  Delay14/1 -> Cell3/1(X_in_0)
  Delay15/1 -> Cell3/2(Y_in_0)
  Delay16/1 -> Cell3/3(Ang_in_0)
  Delay12/1 -> Cell2/3(Ang_in_0)
  Delay11/1 -> Cell2/2(Y_in_0)
  Delay10/1 -> Cell2/1(X_in_0)
  Delay6/1 -> Delay13/1
  Cell1/3(Ang_out_0) -> Delay12/1
  Cell1/2(Y_out_0) -> Delay11/1
  Cell1/1(X_out_0) -> Delay10/1
  Delay9/1 -> Cell1/1(X_in_0)
  Delay8/1 -> Cell1/2(Y_in_0)
  Delay7/1 -> Cell1/3(Ang_in_0)
  Delay5/1 -> Delay6/1
  Cell0/3(Ang_out_0) -> Delay7/1
  Cell0/2(Y_out_0) -> Delay8/1
  Cell0/1(X_out_0) -> Delay9/1
  QUAD_MAP/4(QUAD_CTRL_OUT) -> Delay5/1
  Delay3/1 -> Cell0/2(Y_in_0)
  Delay2/1 -> Cell0/1(X_in_0)
  QUAD_MAP/3(ANG_OUT) -> Delay4/1
  QUAD_MAP/2(Yout) -> Delay3/1
  QUAD_MAP/1(Xout) -> Delay2/1
  Delay47/1 -> QUAD_MAP/1(Xin)
  Delay48/1 -> QUAD_MAP/2(Yin)
  GAIN_CORR/1(XOUT) -> Delay86/1
  Complex to Real-Imag/2 -> Data Type Conversion9/1
  DataInRotate/1 -> Complex to Real-Imag/1
  Complex to Real-Imag/1 -> Data Type Conversion8/1
  Delay86/1 -> Real-Imag to Complex/1
  Delay42/1 -> Real-Imag to Complex/2
  Real-Imag to Complex/1 -> "DataOutRotate  "/1

== system OFDM_Rx_HW/OFDMRx/PhaseTracking_1/DataArrange ==
  note: Re-arrange data symbols
  dataIn : Inport
  dataValidIn : Inport  Port=2
  Delay : Delay  DelayLength=64  InitialCondition=0  UseCircularBuffer=on
  Delay3 : Delay  DelayLength=1  InitialCondition=0  UseCircularBuffer=on
  Dual Port RAM : hdlsllib/HDL RAMs/Dual Port RAM  ram_size=7
      settings: SourceProductBaseCode=SL
  HDL Counter : hdlsllib/Sources/HDL Counter  CountType=Count limited  CountInit=0  CountStep=1  CountMax=127  CountFromType=Initial value  CountFrom=0  CountResetPort=off  CountLoadPort=off  CountEnbPort=on  CountDirPort=off  CountDataType=Unsigned  CountWordLen=7  CountFracLen=0  CountSampTime=1
  HDL Counter1 : hdlsllib/Sources/HDL Counter  CountType=Count limited  CountInit=0  CountStep=1  CountMax=127  CountFromType=Initial value  CountFrom=0  CountResetPort=off  CountLoadPort=off  CountEnbPort=on  CountDirPort=off  CountDataType=Unsigned  CountWordLen=7  CountFracLen=0  CountSampTime=1
  READ_ADDRESS : Lookup_n-D  NumberOfTableDimensions=1  LookupTableObject=''  BreakpointsForDimension1=[0:127]  BreakpointsForDimension1FirstPoint=10  BreakpointsForDimension2FirstPoint=10  BreakpointsForDimension1Spacing=12  BreakpointsForDimension2Spacing=12  IndexSearchMethod=Evenly spaced points  Table=read_addr_rx  TableDataTypeStr=fixdt(0,7,0)  InterpMethod=Flat  DiagnosticForOutOfRangeInput=Error  InternalRulePriority=Speed  OutDataTypeStr=fixdt(0,7,0)  RndMeth=Simplest  InputSameDT=on
  READ_CTRL : Subsystem
  Terminator : Terminator
  dataValidGen : Subsystem
  dataOut : Outport  VectorParamsAs1DForOutWhenUnconnected=off
  dataValidOut : Outport  Port=2  VectorParamsAs1DForOutWhenUnconnected=off
  wires:
  Dual Port RAM/1 -> Terminator/1
  dataValidIn/1 -> Delay/1, HDL Counter1/1, Dual Port RAM/3
  HDL Counter/1 -> READ_ADDRESS/1
  Dual Port RAM/2 -> dataOut/1
  dataIn/1 -> Dual Port RAM/1
  HDL Counter1/1 -> Dual Port RAM/2
  Delay/1 -> HDL Counter/1, Delay3/1, READ_CTRL/2(In2)
  READ_CTRL/1(Out1) -> Dual Port RAM/4
  READ_ADDRESS/1 -> READ_CTRL/1(In1)
  Delay3/1 -> dataValidGen/1(enb)
  dataValidGen/1(dataValidOut) -> dataValidOut/1
